simulink model "soft_real_time_block"  (R2016b)
settings: Solver=FixedStepAuto  StartTime=0.0  StopTime=36000  FixedStep=h_fixed  RelTol=1e-3
libraries: simulink x1
settings Model: Creator=comperem  LastModifiedBy=comperem

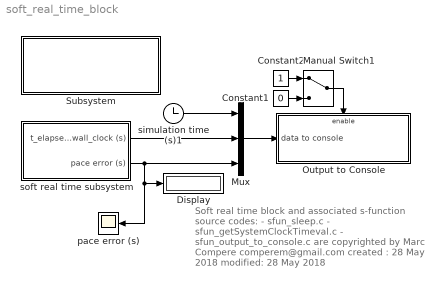
== system soft_real_time_block ==
  note: Soft real time block and associated
      | s-function source codes:
      | - sfun_sleep.c
      | - sfun_getSystemClockTimeval.c
      | - sfun_output_to_console.c
      | are copyrighted
      | by Marc Compere
      | comperem@gmail.com
      | created : 28 May 2018
      | modified: 28 May 2018
  Constant1 : Constant  Value=0
  Constant2 : Constant
  Display : Display
  Manual Switch1 : ManualSwitch
  Mux : Mux  Inputs=3
  Output to Console : Subsystem  TreatAsAtomicUnit=on
  Subsystem : Subsystem
      settings: OpenFcn=h_fixed=0.001
      mask Display: fprintf('Double-Click to init\nstepsize variable, h_fixed')
  "pace error (s) " : Scope
  simulation time (s)1 : Clock
  soft real time subsystem : Subsystem  mask{t_sample=0.01}
      mask prompts: t_sample "Sleep function interval (s)"
  wires:
  Constant2/1 -> Manual Switch1/1
  Constant1/1 -> Manual Switch1/2
  Manual Switch1/1 -> Output to Console/Enable
  Mux/1 -> Output to Console/1(data to console)
  simulation time (s)1/1 -> Mux/1
  soft real time subsystem/1(t_elapsed_wall_clock (s)) -> Mux/2
  soft real time subsystem/2(pace error (s)) -> "pace error (s) "/1, Display/1, Mux/3

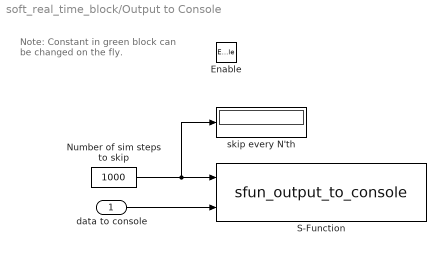
== system soft_real_time_block/Output to Console ==
  note: Note: Constant in green block
      |           can be changed on the fly.
  data to console : Inport
  Enable : EnablePort
  Number of sim steps to skip : Constant  Value=1000
  S-Function : S-Function  FunctionName=sfun_output_to_console  Parameters='[tSimElapsed, tWallElapsed, absTimeErr (s)]: '  SFunctionDeploymentMode=off  EnableBusSupport=off
  skip every N'th : Display
  wires:
  Number of sim steps to skip/1 -> S-Function/1, skip every N'th/1
  data to console/1 -> S-Function/2

== system soft_real_time_block/Subsystem ==

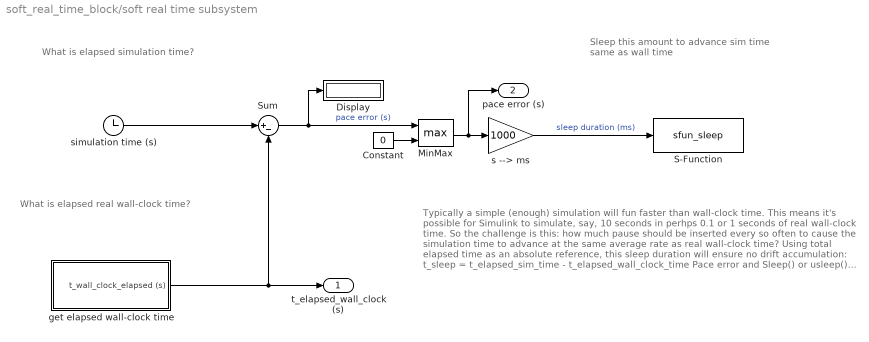
== system soft_real_time_block/soft real time subsystem ==
  note: What is elapsed real
      | wall-clock time?
  note: What is elapsed
      | simulation time?
  note: Sleep this amount
      | to advance sim time
      | same as wall time
  note: Typically a simple (enough) simulation will fun faster than
      | wall-clock time. This means it's possible for Simulink to
      | simulate, say, 10 seconds in perhps 0.1 or 1 seconds of real
      | wall-clock time.
      |
      | So the challenge is this: how much pause should be inserted
      | every so often to cause the simulation time to advance at
      | the same average rate as real wall-clock time?
      |
      | Using total elapsed time as an absolute reference, this
      | sleep duration will ensure no drift accumulation:
      |
      |      t_sleep = t_elapsed_sim_time - t_elapsed_wall_clock_time
      |
      | Pace error and Sleep() or usleep() resolution is system dependent
      | and likely around 10ms on Windows machines. Better on linux.
      |
      | Marc Compere
      | comperem@gmail.com
      | created : 28 May 2018
      | modified: 29 May 2018
  Constant : Constant  Value=0
  Display : Display
  MinMax : MinMax  Function=max  Inputs=2
  S-Function : S-Function  FunctionName=sfun_sleep  Parameters=t_sample  SFunctionDeploymentMode=off  EnableBusSupport=off
  Sum : Sum  Inputs=|+-
  get elapsed wall-clock time : Subsystem
  s --> ms : Gain  Gain=1000
  simulation time (s) : Clock
  t_elapsed_wall_clock (s) : Outport
  pace error (s) : Outport  Port=2
  wires:
  simulation time (s)/1 -> Sum/1
  Constant/1 -> MinMax/2
  get elapsed wall-clock time/1(t_wall_clock_elapsed (s)) -> t_elapsed_wall_clock (s)/1, Sum/2
  Sum/1 -> Display/1, MinMax/1  "pace error (s)"
  MinMax/1 -> pace error (s)/1, s --> ms/1
  s --> ms/1 -> S-Function/1  "sleep duration (ms)"

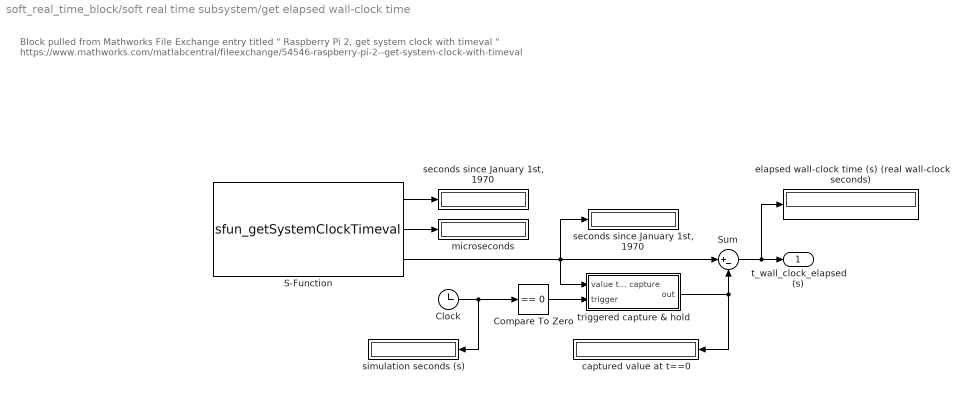
== system soft_real_time_block/soft real time subsystem/get elapsed wall-clock time ==
  note: Block pulled from Mathworks File Exchange entry titled " Raspberry Pi 2, get system clock with timeval "
      |
      | https://www.mathworks.com/matlabcentral/fileexchange/54546-raspberry-pi-2--get-system-clock-with-timeval
  Clock : Clock
  Compare To Zero : simulink/Logic and Bit Operations/Compare To Zero  relop===  OutDataTypeStr=boolean
  S-Function : S-Function  FunctionName=sfun_getSystemClockTimeval  SFunctionDeploymentMode=off  EnableBusSupport=off
  Sum : Sum  Inputs=|+-
  captured value at t==0 : Display
  elapsed wall-clock time (s) (real wall-clock seconds) : Display
  microseconds : Display
  "seconds since January 1st, 1970" : Display
  "seconds since January 1st, 1970 " : Display
  simulation seconds (s) : Display
  triggered capture & hold : Subsystem
  t_wall_clock_elapsed (s) : Outport
  wires:
  triggered capture & hold/1(out) -> captured value at t==0/1, Sum/2
  S-Function/1 -> "seconds since January 1st, 1970 "/1
  Compare To Zero/1 -> triggered capture & hold/2(trigger)
  Sum/1 -> t_wall_clock_elapsed (s)/1, elapsed wall-clock time (s) (real wall-clock seconds)/1
  S-Function/2 -> microseconds/1
  S-Function/3 -> triggered capture & hold/1(value to capture), Sum/1, "seconds since January 1st, 1970"/1
  Clock/1 -> Compare To Zero/1, simulation seconds (s)/1

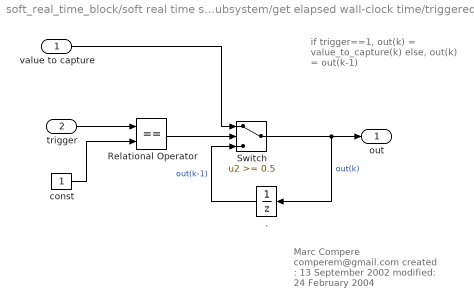
== system soft_real_time_block/soft real time subsystem/get elapsed wall-clock time/triggered capture & hold ==
  note: Marc Compere
      | comperem@gmail.com
      | created  : 13 September 2002
      | modified: 24 February 2004
  note: if trigger==1,
      |    out(k) = value_to_capture(k)
      | else,
      |    out(k) = out(k-1)
  value to capture : Inport
  trigger : Inport  Port=2
  . : UnitDelay  SampleTime=-1
  Relational Operator : RelationalOperator  Operator===  RndMeth=Nearest
  Switch : Switch  Threshold=0.5  SaturateOnIntegerOverflow=on
  const : Constant
  out : Outport
  wires:
  trigger/1 -> Relational Operator/1
  const/1 -> Relational Operator/2
  Relational Operator/1 -> Switch/2
  Switch/1 -> ./1, out/1  "out(k)"
  value to capture/1 -> Switch/1
  ./1 -> Switch/3  "out(k-1)"
